simulink model "setpoint_model"  (R2015b)
settings: Solver=FixedStepDiscrete  StartTime=0.0  StopTime=inf  FixedStep=.001  RelTol=1e-3
libraries: xpcethercatlib x6, slrtlib x2
settings Model: xpc_rtwmakecfg_data=_xpcethercatlib_  SimulationMode=external  Creator=rtheyyun  LastModifiedBy=tech
settings SolverCC: EnableConcurrentExecution=on  ConcurrentTasks=on
settings DataIOCC: SaveFinalState=on  SaveFormat=StructureWithTime  SignalLoggingSaveFormat=ModelDataLogs  InspectSignalLogs=on
settings OptimizationCC: BlockReduction=off  OptimizeBlockIOStorage=off  BufferReuse=off  GlobalBufferReuse=off  ExpressionFolding=off  ExpressionDepthLimit=2147483647  LocalBlockOutputs=off
settings DebuggingCC: ReadBeforeWriteMsg=DisableAll  WriteAfterWriteMsg=DisableAll  WriteAfterReadMsg=DisableAll  UnderspecifiedInitializationDetection=Classic  MergeDetectMultiDrivingBlocksExec=none  SolverPrmCheckMsg=warning  InheritedTsInSrcMsg=none  FcnCallInpInsideContextMsg=UseLocalSettings  StateNameClashWarn=warning
settings HardwareCC: ProdBitPerPointer=32  ProdLargestAtomicFloat=None  ProdWordSize=32  ProdLongLongMode=on  ProdHWDeviceType=Generic->32-bit x86 compatible
settings RTWCC: SystemTargetFile=slrt.tlc  TemplateMakefile=slrt_default_tmf  Description=Simulink Real-Time  RTWVerbose=off  RTWCompilerOptimization=on
settings SimulinkRealTimeCC: GeneratePreprocessorConditionals=Disable all  xPCisModelTimeout=off  xPCModelTimeoutSecs=20  xPCConcurrentTasks=on
settings ConfigComp: CovModelRefEnable=Off  CovSFcnEnable=off

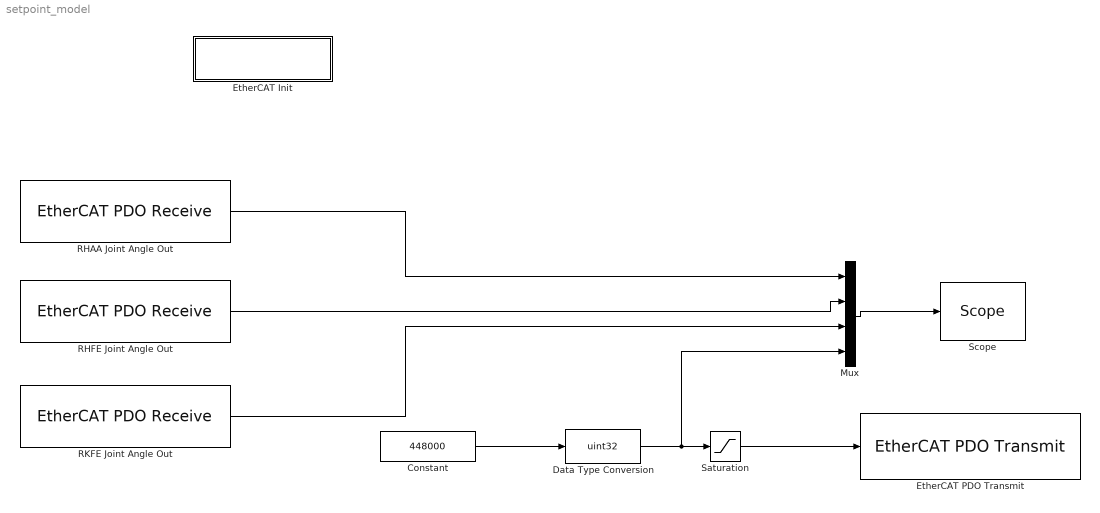
== system setpoint_model ==
  Constant : Constant  Value=448000
  Data Type Conversion : DataTypeConversion  OutDataTypeStr=uint32
  EtherCAT Init : Subsystem
  "EtherCAT PDO Transmit " : xpcethercatlib/EtherCAT PDO Transmit   Priority=3  sig_name=RHAA.Outputs.positionSetpoint  sig_offset=208  sig_type=uint32  type_size=32  sig_dim=1  device_id=0  sample_time=0.010000
  Mux : Mux
  RHAA Joint Angle Out : xpcethercatlib/EtherCAT PDO Receive  Priority=2  sig_name=RHAA.Inputs.jointAngle  sig_offset=208  sig_type=uint32  type_size=32  sig_dim=1  device_id=0  sample_time=0.010000
  RHFE Joint Angle Out : xpcethercatlib/EtherCAT PDO Receive  Priority=2  sig_name=RHAA.Inputs.jointAngle  sig_offset=208  sig_type=uint32  type_size=32  sig_dim=1  device_id=0  sample_time=0.010000
  RKFE Joint Angle Out : xpcethercatlib/EtherCAT PDO Receive  Priority=2  sig_name=RHAA.Inputs.jointAngle  sig_offset=208  sig_type=uint32  type_size=32  sig_dim=1  device_id=0  sample_time=0.010000
  Saturation : Saturate  UpperLimit=468630  LowerLimit=438043
  "Scope " : slrtlib/Displays and Logging/Scope   scopeno=2  scopetype=Target  autostart=on  viewmode=Numerical  formatstr='%15.6f'  grid=on  ylimits=[0,0]  nosamples=3  noprepostsamples=0  interleave=1  triggermode=FreeRun  triggersignal=1  trigsignalfromport=off  triggerlevel=0.0  triggerslope=Either  triggerscope=1  triggersample=0  filename=data.dat  mode=Lazy  writesize=512  autorestart=off  dynamicfilemode=off  maxwritefilesize=512*1024^2
  wires:
  Mux/1 -> "Scope "/1
  RHAA Joint Angle Out/1 -> Mux/1
  RHFE Joint Angle Out/1 -> Mux/2
  RKFE Joint Angle Out/1 -> Mux/3
  Saturation/1 -> "EtherCAT PDO Transmit "/1
  Constant/1 -> Data Type Conversion/1
  Data Type Conversion/1 -> Mux/4, Saturation/1

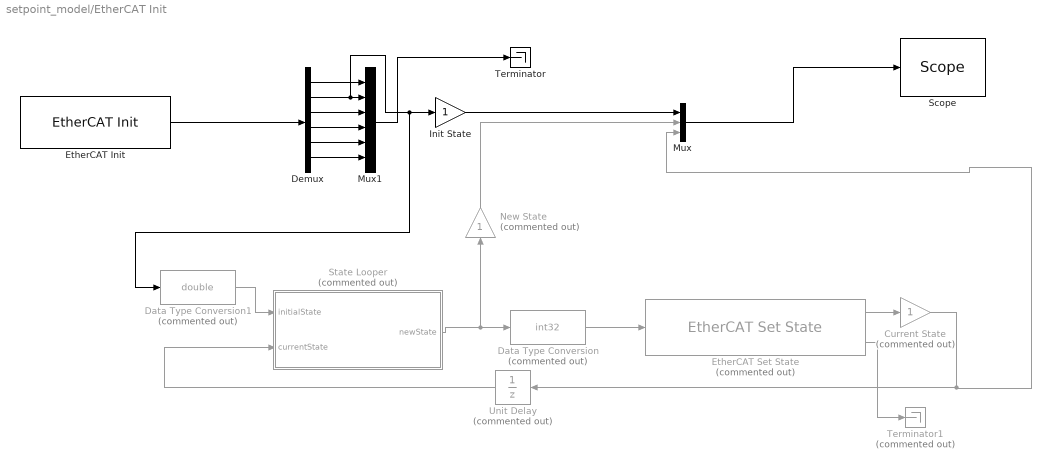
== system setpoint_model/EtherCAT Init ==
  Current State : Gain  Commented=on  OutDataTypeStr=int32
  Data Type Conversion : DataTypeConversion  Commented=on  OutDataTypeStr=int32
  Data Type Conversion1 : DataTypeConversion  Commented=on  OutDataTypeStr=double
  Demux : Demux  Outputs=6
  "EtherCAT Init " : xpcethercatlib/EtherCAT Init   Priority=0  config_file=C:\Software\Simulink Realtime\EtherCAT Config files\single_controller_v1.0.xml  device_id=0  pci_bus=2  pci_slot=0  dctuning=0  enaDebug=off  enaDC=on  errLink=off  masterDbg=off  stateChgDbg=off  baseClock=off  masterCfg=off  logFile='c:\dbglog.txt'  sample_time=0.010000
  "EtherCAT Set State " : xpcethercatlib/EtherCAT Set State   Commented=on  device_id=0  timeout=0  sample_time=0
  Init State : Gain  OutDataTypeStr=int32
  Mux : Mux  Inputs=3
  Mux1 : Mux  Inputs=6
  New State : Gain  Commented=on  OutDataTypeStr=int32
  "Scope " : slrtlib/Displays and Logging/Scope   scopeno=1  scopetype=Target  autostart=on  viewmode=Numerical  formatstr='%15.6f'  grid=on  ylimits=[0,0]  nosamples=3  noprepostsamples=0  interleave=1  triggermode=FreeRun  triggersignal=1  trigsignalfromport=off  triggerlevel=0.0  triggerslope=Either  triggerscope=1  triggersample=0  filename=data.dat  mode=Lazy  writesize=512  autorestart=off  dynamicfilemode=off  maxwritefilesize=512*1024^2
  State Looper : MATLAB Function  Commented=on  TreatAsAtomicUnit=on
  Terminator : Terminator
  Terminator1 : Terminator  Commented=on
  Unit Delay : UnitDelay  Commented=on  SampleTime=-1
  wires:
  Data Type Conversion/1 -> "EtherCAT Set State "/1
  "EtherCAT Set State "/1 -> Current State/1
  "EtherCAT Init "/1 -> Demux/1
  Unit Delay/1 -> State Looper/2(currentState)
  Data Type Conversion1/1 -> State Looper/1(initialState)
  Mux/1 -> "Scope "/1
  Demux/2 -> Mux1/2, Data Type Conversion1/1, Init State/1
  Current State/1 -> Mux/3, Unit Delay/1
  New State/1 -> Mux/2
  State Looper/1(newState) -> Data Type Conversion/1, New State/1
  Init State/1 -> Mux/1
  Demux/1 -> Mux1/1
  Demux/3 -> Mux1/3
  Demux/4 -> Mux1/4
  "EtherCAT Set State "/2 -> Terminator1/1
  Demux/5 -> Mux1/5
  Demux/6 -> Mux1/6
  Mux1/1 -> Terminator/1

== matlab function setpoint_model/EtherCAT Init/State Looper ==
  data: initialState input; newState output; currentState input
function newState = fcn(initialState, currentState)

states = [1 2 4 8];
newState = 8;
if(initialState >= 1 && initialState ~= 8)

    for i = 1 : length(states)
        if(states(i) == currentState && i < 4)
            newState = states(i+1);
        end
    end
else
    newState = initialState;
end
